simulink model "chap05"  (R2021a)
settings: Solver=FixedStepDiscrete  StartTime=0.0  StopTime=inf  FixedStep=0.001  RelTol=1e-3
undefined symbols (not defined in the file): DiscIntNeverNeededParam, Header, Pose, X, Y, Z
libraries: robotlib x31
(part 2 of 9)

== system chap05/Subsystem16/Subsystem1 ==
  In19 : Inport
  switch : Inport  Port=2
  Bus Creator : BusCreator  Inputs=3
  Bus Selector : BusSelector  OutputSignals=state(tk).node5.xx,state(tk).node5.xx0,state(tk).node3.xx,state(tk).node4.xx,state(tk).node5.vx,state(tk).node5.vx0,state(tk).node3.vx,state(tk).node4.vx
  Bus Selector1 : BusSelector  OutputSignals=state(tk).node5.xy,state(tk).node5.xy0,state(tk).node3.xy,state(tk).node4.xy,state(tk).node5.vy,state(tk).node5.vy0,state(tk).node3.vy,state(tk).node4.vy
  Bus Selector2 : BusSelector  OutputSignals=state(tk).node5.xz,state(tk).node5.xz0,state(tk).node3.xz,state(tk).node4.xz,state(tk).node5.vz,state(tk).node5.vz0,state(tk).node3.vz,state(tk).node4.vz
  Bus Selector3 : BusSelector  OutputSignals=state(t).node5.vx,state(t).node0.vx
  Bus Selector4 : BusSelector  OutputSignals=state(t).node5.vy,state(t).node0.vx
  Bus Selector5 : BusSelector  OutputSignals=state(t).node5.vz,state(t).node0.vz
  Bus Selector6 : BusSelector  OutputSignals=state(t).node5.vx,state(t).node5.vy,state(t).node5.vz
  Bus Selector7 : BusSelector  OutputSignals=state(t).node5.vx,state(t).node5.vy,state(t).node5.vz
  Bus Selector8 : BusSelector  OutputSignals=control.node5.ux,control.node5.uy,control.node5.uz
  Subsystem1 : Subsystem
  Subsystem10 : Subsystem
  Subsystem11 : Subsystem
      settings: PortSchema="{\"entries\":[{\"content\":{\"sides\":[{\"content\":{\"connectorIds\":[\"In1\",\"In2\",\"In3\",\"In4\"]},\"type\":\"ConnectorPlacement.EquallySpacedRectSide\",\"uuid\":\"3c32f130-2df4-4697-80e9-267a8217898e\"},{\"content\":{\"connectorIds\":[\"Out1\"],\"side\":\"RIGHT\"},\"type\":\"ConnectorPlacement.EquallySpacedRectSide\",\"uuid\":\"840675a7-4714-440f-a6ce-75eff1b2763f\"},{\"content\":{\"connectorIds\":[\"In5\"],\"side\":\"TOP\"},\"type\":\"ConnectorPlacement.EquallySpacedRectSide\",\"uuid\":\"5c23af56-4ec3-4a39-a531-12998a0be3c8\"},{\"content\":{\"connectorIds\":[\"Out2\"],\"side\":\"BOTTOM\"},\"type\":\"ConnectorPlacement.EquallySpacedRectSide\",\"uuid\":\"31d953fb-65a0-42e9-a844-060de010f298\"}]},\"type\":\"ConnectorPlacement.EquallySpacedConnector\",\"uuid\":\"61b27aa3-5880-401e-bae3-4611093a191a\"}],\"packageUris\":[\"http://schema.mathworks.com/mf0/Connector/R2020b\"],\"version\":\"1.0\"}"
  Subsystem2 : Subsystem
  Subsystem3 : Subsystem
      settings: PortSchema="{\"entries\":[{\"content\":{\"sides\":[{\"content\":{\"connectorIds\":[\"In1\",\"In2\",\"In3\",\"In4\",\"In5\",\"In6\",\"In7\",\"In8\",\"In9\"]},\"type\":\"ConnectorPlacement.EquallySpacedRectSide\",\"uuid\":\"e02b19dc-feca-4a5f-b0a9-7b682689d3dc\"},{\"content\":{\"connectorIds\":[\"Out1\",\"Out2\",\"Out3\"],\"side\":\"RIGHT\"},\"type\":\"ConnectorPlacement.EquallySpacedRectSide\",\"uuid\":\"6cba16a1-1866-4332-a766-c6ecae75c00a\"},{\"content\":{\"connectorIds\":[],\"side\":\"TOP\"},\"type\":\"ConnectorPlacement.EquallySpacedRectSide\",\"uuid\":\"834934d8-ba7c-4cfc-8528-dda956d123e9\"},{\"content\":{\"connectorIds\":[\"In10\"],\"side\":\"BOTTOM\"},\"type\":\"ConnectorPlacement.EquallySpacedRectSide\",\"uuid\":\"a447ec2e-850c-49d1-98c5-4201d925b22c\"}]},\"type\":\"ConnectorPlacement.EquallySpacedConnector\",\"uuid\":\"dde62e81-0b86-43c6-8cdc-67ebf109c079\"}],\"packageUris\":[\"http://schema.mathworks.com/mf0/Connector/R2020b\"],\"version\":\"1.0\"}"
  Subsystem5 : Subsystem
      settings: PortSchema="{\"entries\":[{\"content\":{\"sides\":[{\"content\":{\"connectorIds\":[\"In1\",\"In2\",\"In3\",\"In4\"]},\"type\":\"ConnectorPlacement.EquallySpacedRectSide\",\"uuid\":\"3c32f130-2df4-4697-80e9-267a8217898e\"},{\"content\":{\"connectorIds\":[\"Out1\"],\"side\":\"RIGHT\"},\"type\":\"ConnectorPlacement.EquallySpacedRectSide\",\"uuid\":\"840675a7-4714-440f-a6ce-75eff1b2763f\"},{\"content\":{\"connectorIds\":[\"In5\"],\"side\":\"TOP\"},\"type\":\"ConnectorPlacement.EquallySpacedRectSide\",\"uuid\":\"5c23af56-4ec3-4a39-a531-12998a0be3c8\"},{\"content\":{\"connectorIds\":[\"Out2\"],\"side\":\"BOTTOM\"},\"type\":\"ConnectorPlacement.EquallySpacedRectSide\",\"uuid\":\"31d953fb-65a0-42e9-a844-060de010f298\"}]},\"type\":\"ConnectorPlacement.EquallySpacedConnector\",\"uuid\":\"61b27aa3-5880-401e-bae3-4611093a191a\"}],\"packageUris\":[\"http://schema.mathworks.com/mf0/Connector/R2020b\"],\"version\":\"1.0\"}"
  Subsystem6 : Subsystem
  Subsystem8 : Subsystem
      settings: PortSchema="{\"entries\":[{\"content\":{\"sides\":[{\"content\":{\"connectorIds\":[\"In1\",\"In2\",\"In3\",\"In4\",\"In5\",\"In6\"]},\"type\":\"ConnectorPlacement.EquallySpacedRectSide\",\"uuid\":\"6e2ae49e-f829-4a88-ba6d-12a1c984ff97\"},{\"content\":{\"connectorIds\":[\"Out1\"],\"side\":\"RIGHT\"},\"type\":\"ConnectorPlacement.EquallySpacedRectSide\",\"uuid\":\"1d02df48-94d5-4b75-9fdc-37bb62799324\"},{\"content\":{\"connectorIds\":[],\"side\":\"TOP\"},\"type\":\"ConnectorPlacement.EquallySpacedRectSide\",\"uuid\":\"e0c2a01b-94eb-432a-818f-b3ac4af71c3e\"},{\"content\":{\"connectorIds\":[\"In7\"],\"side\":\"BOTTOM\"},\"type\":\"ConnectorPlacement.EquallySpacedRectSide\",\"uuid\":\"1c8c54e5-1608-4962-a210-31f0a1951aa9\"}]},\"type\":\"ConnectorPlacement.EquallySpacedConnector\",\"uuid\":\"4e183442-7783-4f10-aa1a-c21f2f9b268a\"}],\"packageUris\":[\"http://schema.mathworks.com/mf0/Connector/R2020b\"],\"version\":\"1.0\"}"
  Subsystem9 : Subsystem
      settings: PortSchema="{\"entries\":[{\"content\":{\"sides\":[{\"content\":{\"connectorIds\":[\"In1\",\"In2\",\"In3\",\"In4\"]},\"type\":\"ConnectorPlacement.EquallySpacedRectSide\",\"uuid\":\"3c32f130-2df4-4697-80e9-267a8217898e\"},{\"content\":{\"connectorIds\":[\"Out1\"],\"side\":\"RIGHT\"},\"type\":\"ConnectorPlacement.EquallySpacedRectSide\",\"uuid\":\"840675a7-4714-440f-a6ce-75eff1b2763f\"},{\"content\":{\"connectorIds\":[\"In5\"],\"side\":\"TOP\"},\"type\":\"ConnectorPlacement.EquallySpacedRectSide\",\"uuid\":\"5c23af56-4ec3-4a39-a531-12998a0be3c8\"},{\"content\":{\"connectorIds\":[\"Out2\"],\"side\":\"BOTTOM\"},\"type\":\"ConnectorPlacement.EquallySpacedRectSide\",\"uuid\":\"31d953fb-65a0-42e9-a844-060de010f298\"}]},\"type\":\"ConnectorPlacement.EquallySpacedConnector\",\"uuid\":\"61b27aa3-5880-401e-bae3-4611093a191a\"}],\"packageUris\":[\"http://schema.mathworks.com/mf0/Connector/R2020b\"],\"version\":\"1.0\"}"
  u5 : Outport
  wires:
  Bus Creator/1 -> u5/1  "node5"
  Bus Selector/5 -> Subsystem6/5(vx5)  "<vx>"
  Bus Selector/1 -> Subsystem6/1(xx5)  "<xx>"
  Bus Selector/3 -> Subsystem6/3(xx3)  "<xx>"
  Bus Selector/8 -> Subsystem6/8(vx4)  "<vx>"
  Bus Selector/7 -> Subsystem6/7(vx3)  "<vx>"
  Bus Selector/4 -> Subsystem6/4(xx4)  "<xx>"
  Bus Selector6/3 -> Subsystem8/6(vz)  "<vz>"
  Bus Selector6/1 -> Subsystem8/4(vx)  "<vx>"
  [Sx] -> Subsystem8/1(Sx)
  [Sz] -> Subsystem8/3(Sz)
  Subsystem8/1(" gain") -> [gain]  "p5"
  In19/1 -> [state], Bus Selector2/1, Bus Selector/1, Bus Selector1/1
  [state] -> Bus Selector6/1
  [Sy] -> Subsystem8/2(Sy)
  Bus Selector6/2 -> Subsystem8/5(vy)  "<vy>"
  Subsystem10/3(uz) -> Bus Creator/3  "uz"
  Subsystem10/2(uy) -> Bus Creator/2  "uy"
  Subsystem10/1(ux) -> Bus Creator/1  "ux"
  [state] -> Bus Selector7/1
  Bus Selector8/1 -> Subsystem3/6(ux)  "<ux>"
  Bus Selector7/2 -> Subsystem3/3(vy)  "<vy>"
  Bus Selector8/2 -> Subsystem3/7(uy)  "<uy>"
  [state] -> Bus Selector8/1
  Bus Selector7/1 -> Subsystem3/2(vx)  "<vx>"
  Bus Selector7/3 -> Subsystem3/4(vz)  "<vz>"
  Bus Selector8/3 -> Subsystem3/8(uz)  "<uz>"
  Subsystem3/1(udtx) -> Subsystem10/1(utx)
  Subsystem3/2(udty) -> Subsystem10/2(uty)
  Subsystem3/3(udtz) -> Subsystem10/3(utz)
  Bus Selector/2 -> Subsystem6/2(xx0)  "<xx0>"
  Bus Selector/6 -> Subsystem6/6(vx0)  "<vx0>"
  Bus Selector1/1 -> Subsystem1/1(xy5)  "<xy>"
  Bus Selector1/2 -> Subsystem1/2(xy0)  "<xy0>"
  Bus Selector1/3 -> Subsystem1/3(xy3)  "<xy>"
  Bus Selector1/4 -> Subsystem1/4(xy4)  "<xy>"
  Bus Selector1/5 -> Subsystem1/5(vy5)  "<vy>"
  Bus Selector1/6 -> Subsystem1/6(vy0)  "<vy0>"
  Bus Selector1/7 -> Subsystem1/7(vy3)  "<vy>"
  Bus Selector1/8 -> Subsystem1/8(vy4)  "<vy>"
  Bus Selector2/1 -> Subsystem2/1(xz5)  "<xz>"
  Bus Selector2/2 -> Subsystem2/2(xz0)  "<xz0>"
  Bus Selector2/3 -> Subsystem2/3(xz3)  "<xz>"
  Bus Selector2/4 -> Subsystem2/4(xz4)  "<xz>"
  Bus Selector2/5 -> Subsystem2/5(vz5)  "<vz>"
  Bus Selector2/6 -> Subsystem2/6(vz0)  "<vz0>"
  Bus Selector2/7 -> Subsystem2/7(vz3)  "<vz>"
  Bus Selector2/8 -> Subsystem2/8(vz4)  "<vz>"
  [gain] -> Subsystem11/4(gain)
  Subsystem9/1(uy) -> Subsystem3/5(uty)
  Subsystem2/1(utz) -> Subsystem11/3(utz)
  Subsystem1/1(uty) -> Subsystem9/3(uty)
  [state] -> Bus Selector3/1
  Subsystem5/1(ux) -> Subsystem3/1(utx)
  Bus Selector3/2 -> Subsystem5/2(vx0)  "<vx>"
  Bus Selector3/1 -> Subsystem5/1(vx5)  "<vx>"
  Subsystem11/1(uz) -> Subsystem3/9(utz)
  Bus Selector5/1 -> Subsystem11/1(vz5)  "<vz>"
  [state] -> Bus Selector4/1
  Subsystem6/1(utx) -> Subsystem5/3(utx)
  [state] -> Bus Selector5/1
  Bus Selector4/1 -> Subsystem9/1(vy5)  "<vy>"
  Bus Selector4/2 -> Subsystem9/2(vy0)  "<vx>"
  Bus Selector5/2 -> Subsystem11/2(vz0)  "<vz>"
  [gain] -> Subsystem5/4(gain)
  Subsystem5/2(Sx) -> [Sx]
  Subsystem9/2(Sz) -> [Sy]
  Subsystem11/2(Sz) -> [Sz]
  [gain] -> Subsystem9/4(gain)
  switch/1 -> [switch], Subsystem5/5(switch)
  [switch] -> Subsystem11/5(switch)
  [switch] -> Subsystem9/5(switch)
  [switch] -> Subsystem8/7(switch)
  [switch] -> Subsystem3/10(switch)

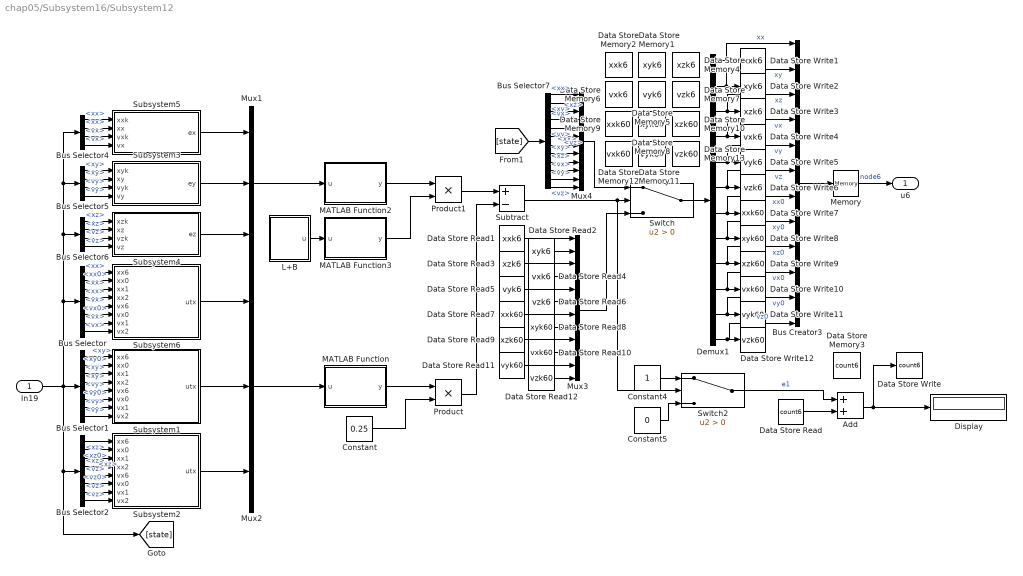
== system chap05/Subsystem16/Subsystem12 ==
  In19 : Inport
  Add : Sum
  Bus Creator3 : BusCreator  Inputs=12
  Bus Selector : BusSelector  OutputSignals=state(tk).node6.xx,state(tk).node6.xx0,state(tk).node1.xx,state(tk).node2.xx,state(tk).node6.vx,state(tk).node6.vx0,state(tk).node1.vx,state(tk).node2.vx
  Bus Selector1 : BusSelector  OutputSignals=state(tk).node6.xy,state(tk).node6.xy0,state(tk).node1.xy,state(tk).node2.xy,state(tk).node6.vy,state(tk).node6.vy0,state(tk).node1.vy,state(tk).node2.vy
  Bus Selector2 : BusSelector  OutputSignals=state(tk).node6.xz,state(tk).node6.xz0,state(tk).node1.xz,state(tk).node2.xz,state(tk).node6.vz,state(tk).node6.vz0,state(tk).node1.vz,state(tk).node2.vz
  Bus Selector4 : BusSelector  OutputSignals=state(tk).node6.xx,state(t).node6.xx,state(tk).node6.vx,state(t).node6.vx
  Bus Selector5 : BusSelector  OutputSignals=state(tk).node6.xy,state(t).node6.xy,state(tk).node6.vy,state(t).node6.vy
  Bus Selector6 : BusSelector  OutputSignals=state(tk).node6.xz,state(t).node6.xz,state(tk).node6.vz,state(t).node6.vz
  Bus Selector7 : BusSelector  OutputSignals=state(t).node6.xx,state(t).node6.xy,state(t).node6.xz,state(t).node6.vx,state(t).node6.vy,state(t).node6.vz,state(t).node0.xx,state(t).node0.xy,state(t).node0.xz,state(t).node0.vx,state(t).node0.vy,state(t).node0.vz
  Constant : Constant  Value=0.25
  Constant4 : Constant
  Constant5 : Constant  Value=0
  Data Store Memory1 : DataStoreMemory  DataStoreName=xyk6  ReadBeforeWriteMsg=warning  WriteAfterWriteMsg=warning  WriteAfterReadMsg=warning  ShowAdditionalParam=off
  Data Store Memory10 : DataStoreMemory  DataStoreName=xzk60  ReadBeforeWriteMsg=warning  WriteAfterWriteMsg=warning  WriteAfterReadMsg=warning  ShowAdditionalParam=off
  Data Store Memory11 : DataStoreMemory  DataStoreName=vyk60  ReadBeforeWriteMsg=warning  WriteAfterWriteMsg=warning  WriteAfterReadMsg=warning  ShowAdditionalParam=off
  Data Store Memory12 : DataStoreMemory  DataStoreName=vxk60  ReadBeforeWriteMsg=warning  WriteAfterWriteMsg=warning  WriteAfterReadMsg=warning  ShowAdditionalParam=off
  Data Store Memory13 : DataStoreMemory  DataStoreName=vzk60  ReadBeforeWriteMsg=warning  WriteAfterWriteMsg=warning  WriteAfterReadMsg=warning  ShowAdditionalParam=off
  Data Store Memory2 : DataStoreMemory  DataStoreName=xxk6  ReadBeforeWriteMsg=warning  WriteAfterWriteMsg=warning  WriteAfterReadMsg=warning  ShowAdditionalParam=off
  Data Store Memory3 : DataStoreMemory  DataStoreName=count6  ReadBeforeWriteMsg=warning  WriteAfterWriteMsg=warning  WriteAfterReadMsg=warning  ShowAdditionalParam=off
  Data Store Memory4 : DataStoreMemory  DataStoreName=xzk6  ReadBeforeWriteMsg=warning  WriteAfterWriteMsg=warning  WriteAfterReadMsg=warning  ShowAdditionalParam=off
  Data Store Memory5 : DataStoreMemory  DataStoreName=vyk6  ReadBeforeWriteMsg=warning  WriteAfterWriteMsg=warning  WriteAfterReadMsg=warning  ShowAdditionalParam=off
  Data Store Memory6 : DataStoreMemory  DataStoreName=vxk6  ReadBeforeWriteMsg=warning  WriteAfterWriteMsg=warning  WriteAfterReadMsg=warning  ShowAdditionalParam=off
  Data Store Memory7 : DataStoreMemory  DataStoreName=vzk6  ReadBeforeWriteMsg=warning  WriteAfterWriteMsg=warning  WriteAfterReadMsg=warning  ShowAdditionalParam=off
  Data Store Memory8 : DataStoreMemory  DataStoreName=xyk60  ReadBeforeWriteMsg=warning  WriteAfterWriteMsg=warning  WriteAfterReadMsg=warning  ShowAdditionalParam=off
  Data Store Memory9 : DataStoreMemory  DataStoreName=xxk60  ReadBeforeWriteMsg=warning  WriteAfterWriteMsg=warning  WriteAfterReadMsg=warning  ShowAdditionalParam=off
  Data Store Read : DataStoreRead  DataStoreName=count6  IndexOptions=Index vector (dialog)  Indices=1  OutputSizes=1
  Data Store Read1 : DataStoreRead  DataStoreName=xxk6  IndexOptions=Index vector (dialog)  Indices=1  OutputSizes=1
  Data Store Read10 : DataStoreRead  DataStoreName=vxk60  IndexOptions=Index vector (dialog)  Indices=1  OutputSizes=1
  Data Store Read11 : DataStoreRead  DataStoreName=vyk60  IndexOptions=Index vector (dialog)  Indices=1  OutputSizes=1
  Data Store Read12 : DataStoreRead  DataStoreName=vzk60  IndexOptions=Index vector (dialog)  Indices=1  OutputSizes=1
  Data Store Read2 : DataStoreRead  DataStoreName=xyk6  IndexOptions=Index vector (dialog)  Indices=1  OutputSizes=1
  Data Store Read3 : DataStoreRead  DataStoreName=xzk6  IndexOptions=Index vector (dialog)  Indices=1  OutputSizes=1
  Data Store Read4 : DataStoreRead  DataStoreName=vxk6  IndexOptions=Index vector (dialog)  Indices=1  OutputSizes=1
  Data Store Read5 : DataStoreRead  DataStoreName=vyk6  IndexOptions=Index vector (dialog)  Indices=1  OutputSizes=1
  Data Store Read6 : DataStoreRead  DataStoreName=vzk6  IndexOptions=Index vector (dialog)  Indices=1  OutputSizes=1
  Data Store Read7 : DataStoreRead  DataStoreName=xxk60  IndexOptions=Index vector (dialog)  Indices=1  OutputSizes=1
  Data Store Read8 : DataStoreRead  DataStoreName=xyk60  IndexOptions=Index vector (dialog)  Indices=1  OutputSizes=1
  Data Store Read9 : DataStoreRead  DataStoreName=xzk60  IndexOptions=Index vector (dialog)  Indices=1  OutputSizes=1
  Data Store Write : DataStoreWrite  DataStoreName=count6  IndexOptions=Index vector (dialog)  Indices=1  OutputSizes=1
  Data Store Write1 : DataStoreWrite  DataStoreName=xxk6  IndexOptions=Index vector (dialog)  Indices=1  OutputSizes=1
  Data Store Write10 : DataStoreWrite  DataStoreName=vxk60  IndexOptions=Index vector (dialog)  Indices=1  OutputSizes=1
  Data Store Write11 : DataStoreWrite  DataStoreName=vyk60  IndexOptions=Index vector (dialog)  Indices=1  OutputSizes=1
  Data Store Write12 : DataStoreWrite  DataStoreName=vzk60  IndexOptions=Index vector (dialog)  Indices=1  OutputSizes=1
  Data Store Write2 : DataStoreWrite  DataStoreName=xyk6  IndexOptions=Index vector (dialog)  Indices=1  OutputSizes=1
  Data Store Write3 : DataStoreWrite  DataStoreName=xzk6  IndexOptions=Index vector (dialog)  Indices=1  OutputSizes=1
  Data Store Write4 : DataStoreWrite  DataStoreName=vxk6  IndexOptions=Index vector (dialog)  Indices=1  OutputSizes=1
  Data Store Write5 : DataStoreWrite  DataStoreName=vyk6  IndexOptions=Index vector (dialog)  Indices=1  OutputSizes=1
  Data Store Write6 : DataStoreWrite  DataStoreName=vzk6  IndexOptions=Index vector (dialog)  Indices=1  OutputSizes=1
  Data Store Write7 : DataStoreWrite  DataStoreName=xxk60  IndexOptions=Index vector (dialog)  Indices=1  OutputSizes=1
  Data Store Write8 : DataStoreWrite  DataStoreName=xyk60  IndexOptions=Index vector (dialog)  Indices=1  OutputSizes=1
  Data Store Write9 : DataStoreWrite  DataStoreName=xzk60  IndexOptions=Index vector (dialog)  Indices=1  OutputSizes=1
  Demux1 : Demux  Outputs=12
  Display : Display
  L+B : Subsystem
  MATLAB Function : MATLAB Function  TreatAsAtomicUnit=on
  MATLAB Function2 : MATLAB Function  TreatAsAtomicUnit=on
  MATLAB Function3 : MATLAB Function  TreatAsAtomicUnit=on
  Memory : Memory
  Mux1 : Mux  Inputs=3
  Mux2 : Mux  Inputs=3
  Mux3 : Mux  Inputs=12
  Mux4 : Mux  Inputs=12
  Product : Product
  Product1 : Product
  Subsystem1 : Subsystem
  Subsystem2 : Subsystem
  Subsystem3 : Subsystem
  Subsystem4 : Subsystem
  Subsystem5 : Subsystem
  Subsystem6 : Subsystem
  Subtract : Sum  Inputs=+-
  Switch : Switch  Criteria=u2 > Threshold
  Switch2 : Switch  Criteria=u2 > Threshold
  u6 : Outport
  wires:
  Subsystem1/1(utx) -> Mux2/2
  Subsystem6/1(utx) -> Mux2/1
  Subsystem2/1(utx) -> Mux2/3
  Data Store Read/1 -> Add/2
  Subsystem3/1(ey) -> Mux1/2
  MATLAB Function/1(y) -> Product/1
  Mux2/1 -> MATLAB Function/1(u)
  Product1/1 -> Subtract/1
  Add/1 -> Data Store Write/1, Display/1
  Subsystem5/1(ex) -> Mux1/1
  Subsystem4/1(ez) -> Mux1/3
  Mux1/1 -> MATLAB Function2/1(u)
  L+B/1(u) -> MATLAB Function3/1(u)
  MATLAB Function2/1(y) -> Product1/1
  Constant4/1 -> Switch2/1
  Constant/1 -> Product/2
  Constant5/1 -> Switch2/3
  MATLAB Function3/1(y) -> Product1/2
  Switch2/1 -> Add/1  "e1"
  Product/1 -> Subtract/2
  Memory/1 -> u6/1  "node6"
  Bus Selector4/4 -> Subsystem5/4(vx)  "<vx>"
  Bus Selector5/3 -> Subsystem3/3(vyk)  "<vy>"
  Bus Selector5/2 -> Subsystem3/2(xy)  "<xy>"
  Bus Selector4/1 -> Subsystem5/1(xxk)  "<xx>"
  Bus Selector5/4 -> Subsystem3/4(vy)  "<vy>"
  Bus Selector5/1 -> Subsystem3/1(xyk)  "<xy>"
  In19/1 -> Bus Selector1/1, Bus Selector2/1, [state], Bus Selector/1, Bus Selector5/1, Bus Selector4/1, Bus Selector6/1
  Bus Selector4/3 -> Subsystem5/3(vxk)  "<vx>"
  Bus Selector6/2 -> Subsystem4/2(xz)  "<xz>"
  Bus Selector6/3 -> Subsystem4/3(vzk)  "<vz>"
  Bus Selector4/2 -> Subsystem5/2(xx)  "<xx>"
  Bus Selector6/4 -> Subsystem4/4(vz)  "<vz>"
  Bus Selector6/1 -> Subsystem4/1(xzk)  "<xz>"
  Subtract/1 -> Switch/2, Switch2/2
  Demux1/3 -> Data Store Write3/1, Bus Creator3/3  "xz"
  Demux1/12 -> Bus Creator3/12, Data Store Write12/1  "vz0"
  Demux1/9 -> Data Store Write9/1, Bus Creator3/9  "xz0"
  Data Store Read3/1 -> Mux3/3
  Bus Selector7/10 -> Mux4/10  "<vx>"
  Data Store Read2/1 -> Mux3/2
  Mux3/1 -> Switch/3
  Demux1/10 -> Data Store Write10/1, Bus Creator3/10  "vx0"
  Bus Selector7/5 -> Mux4/5  "<vy>"
  Data Store Read6/1 -> Mux3/6
  Data Store Read5/1 -> Mux3/5
  Demux1/5 -> Data Store Write5/1, Bus Creator3/5  "vy"
  Data Store Read1/1 -> Mux3/1
  Demux1/11 -> Data Store Write11/1, Bus Creator3/11  "vy0"
  Demux1/1 -> Data Store Write1/1, Bus Creator3/1  "xx"
  Data Store Read4/1 -> Mux3/4
  [state] -> Bus Selector7/1
  Data Store Read11/1 -> Mux3/11
  Demux1/6 -> Data Store Write6/1, Bus Creator3/6  "vz"
  Bus Selector7/2 -> Mux4/2  "<xy>"
  Bus Selector7/1 -> Mux4/1  "<xx>"
  Bus Selector7/8 -> Mux4/8  "<xy>"
  Data Store Read10/1 -> Mux3/10
  Bus Selector7/4 -> Mux4/4  "<vx>"
  Mux4/1 -> Switch/1
  Data Store Read12/1 -> Mux3/12
  Bus Creator3/1 -> Memory/1
  Bus Selector7/7 -> Mux4/7  "<xx>"
  Bus Selector7/6 -> Mux4/6  "<vz>"
  Demux1/2 -> Data Store Write2/1, Bus Creator3/2  "xy"
  Demux1/4 -> Data Store Write4/1, Bus Creator3/4  "vx"
  Data Store Read9/1 -> Mux3/9
  Bus Selector7/11 -> Mux4/11  "<vy>"
  Bus Selector7/9 -> Mux4/9  "<xz>"
  Demux1/8 -> Data Store Write8/1, Bus Creator3/8  "xy0"
  Demux1/7 -> Data Store Write7/1, Bus Creator3/7  "xx0"
  Bus Selector7/3 -> Mux4/3  "<xz>"
  Data Store Read7/1 -> Mux3/7
  Data Store Read8/1 -> Mux3/8
  Switch/1 -> Demux1/1
  Bus Selector7/12 -> Mux4/12  "<vz>"
  Bus Selector/2 -> Subsystem6/2(xx0)  "<xx0>"
  Bus Selector1/4 -> Subsystem1/4(xx2)  "<xy>"
  Bus Selector/8 -> Subsystem6/8(vx2)  "<vx>"
  Bus Selector1/5 -> Subsystem1/5(vx6)  "<vy>"
  Bus Selector/6 -> Subsystem6/6(vx0)  "<vx0>"
  Bus Selector1/7 -> Subsystem1/7(vx1)  "<vy>"
  Bus Selector1/2 -> Subsystem1/2(xx0)  "<xy0>"
  Bus Selector1/1 -> Subsystem1/1(xx6)  "<xy>"
  Bus Selector2/1 -> Subsystem2/1(xx6)  "<xz>"
  Bus Selector2/6 -> Subsystem2/6(vx0)  "<vz0>"
  Bus Selector2/5 -> Subsystem2/5(vx6)  "<vz>"
  Bus Selector/5 -> Subsystem6/5(vx6)  "<vx>"
  Bus Selector/7 -> Subsystem6/7(vx1)  "<vx>"
  Bus Selector1/8 -> Subsystem1/8(vx2)  "<vy>"
  Bus Selector2/2 -> Subsystem2/2(xx0)  "<xz0>"
  Bus Selector2/4 -> Subsystem2/4(xx2)  "<xz>"
  Bus Selector/4 -> Subsystem6/4(xx2)  "<xx>"
  Bus Selector/1 -> Subsystem6/1(xx6)  "<xx>"
  Bus Selector1/6 -> Subsystem1/6(vx0)  "<vy0>"
  Bus Selector1/3 -> Subsystem1/3(xx1)  "<xy>"
  Bus Selector/3 -> Subsystem6/3(xx1)  "<xx>"
  Bus Selector2/3 -> Subsystem2/3(xx1)  "<xz>"
  Bus Selector2/7 -> Subsystem2/7(vx1)  "<vz>"
  Bus Selector2/8 -> Subsystem2/8(vx2)  "<vz>"

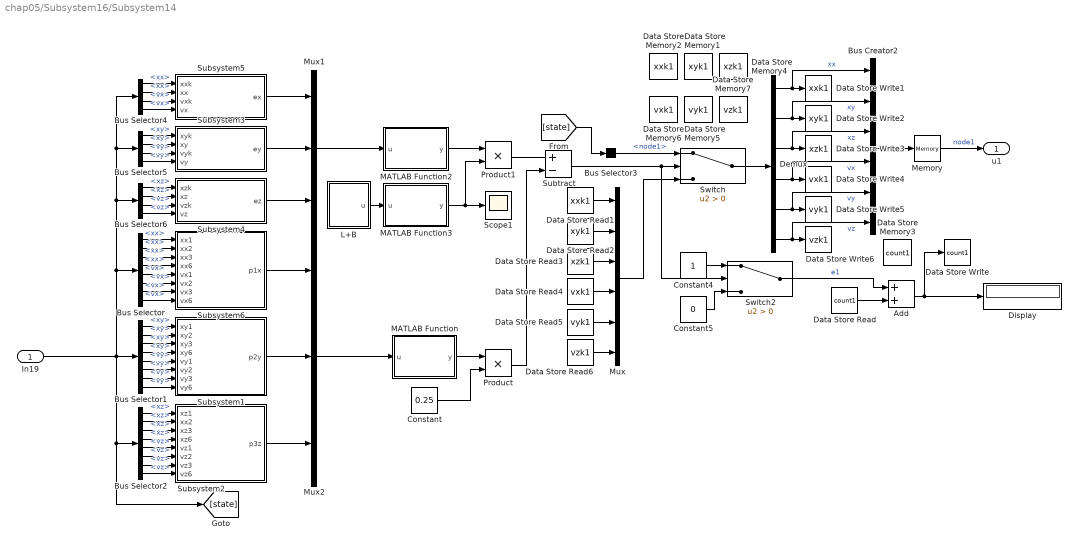
== system chap05/Subsystem16/Subsystem14 ==
  In19 : Inport
  Add : Sum
  Bus Creator2 : BusCreator  Inputs=6
  Bus Selector : BusSelector  OutputSignals=state(tk).node1.xx,state(tk).node2.xx,state(tk).node3.xx,state(tk).node6.xx,state(tk).node1.vx,state(tk).node2.vx,state(tk).node3.vx,state(tk).node6.vx
  Bus Selector1 : BusSelector  OutputSignals=state(tk).node1.xy,state(tk).node2.xy,state(tk).node3.xy,state(tk).node6.xy,state(tk).node1.vy,state(tk).node2.vy,state(tk).node3.vy,state(tk).node6.vy
  Bus Selector2 : BusSelector  OutputSignals=state(tk).node1.xz,state(tk).node2.xz,state(tk).node3.xz,state(tk).node6.xz,state(tk).node1.vz,state(tk).node2.vz,state(tk).node3.vz,state(tk).node6.vz
  Bus Selector3 : BusSelector  OutputSignals=state(t).node1
  Bus Selector4 : BusSelector  OutputSignals=state(tk).node1.xx,state(t).node1.xx,state(tk).node1.vx,state(t).node1.vx
  Bus Selector5 : BusSelector  OutputSignals=state(tk).node1.xy,state(t).node1.xy,state(tk).node1.vy,state(t).node1.vy
  Bus Selector6 : BusSelector  OutputSignals=state(tk).node1.xz,state(t).node1.xz,state(tk).node1.vz,state(t).node1.vz
  Constant : Constant  Value=0.25
  Constant4 : Constant
  Constant5 : Constant  Value=0
  Data Store Memory1 : DataStoreMemory  DataStoreName=xyk1  ReadBeforeWriteMsg=warning  WriteAfterWriteMsg=warning  WriteAfterReadMsg=warning  ShowAdditionalParam=off
  Data Store Memory2 : DataStoreMemory  DataStoreName=xxk1  ReadBeforeWriteMsg=warning  WriteAfterWriteMsg=warning  WriteAfterReadMsg=warning  ShowAdditionalParam=off
  Data Store Memory3 : DataStoreMemory  DataStoreName=count1  ReadBeforeWriteMsg=warning  WriteAfterWriteMsg=warning  WriteAfterReadMsg=warning  ShowAdditionalParam=off
  Data Store Memory4 : DataStoreMemory  DataStoreName=xzk1  ReadBeforeWriteMsg=warning  WriteAfterWriteMsg=warning  WriteAfterReadMsg=warning  ShowAdditionalParam=off
  Data Store Memory5 : DataStoreMemory  DataStoreName=vyk1  ReadBeforeWriteMsg=warning  WriteAfterWriteMsg=warning  WriteAfterReadMsg=warning  ShowAdditionalParam=off
  Data Store Memory6 : DataStoreMemory  DataStoreName=vxk1  ReadBeforeWriteMsg=warning  WriteAfterWriteMsg=warning  WriteAfterReadMsg=warning  ShowAdditionalParam=off
  Data Store Memory7 : DataStoreMemory  DataStoreName=vzk1  ReadBeforeWriteMsg=warning  WriteAfterWriteMsg=warning  WriteAfterReadMsg=warning  ShowAdditionalParam=off
  Data Store Read : DataStoreRead  DataStoreName=count1  IndexOptions=Index vector (dialog)  Indices=1  OutputSizes=1
  Data Store Read1 : DataStoreRead  DataStoreName=xxk1  IndexOptions=Index vector (dialog)  Indices=1  OutputSizes=1
  Data Store Read2 : DataStoreRead  DataStoreName=xyk1  IndexOptions=Index vector (dialog)  Indices=1  OutputSizes=1
  Data Store Read3 : DataStoreRead  DataStoreName=xzk1  IndexOptions=Index vector (dialog)  Indices=1  OutputSizes=1
  Data Store Read4 : DataStoreRead  DataStoreName=vxk1  IndexOptions=Index vector (dialog)  Indices=1  OutputSizes=1
  Data Store Read5 : DataStoreRead  DataStoreName=vyk1  IndexOptions=Index vector (dialog)  Indices=1  OutputSizes=1
  Data Store Read6 : DataStoreRead  DataStoreName=vzk1  IndexOptions=Index vector (dialog)  Indices=1  OutputSizes=1
  Data Store Write : DataStoreWrite  DataStoreName=count1  IndexOptions=Index vector (dialog)  Indices=1  OutputSizes=1
  Data Store Write1 : DataStoreWrite  DataStoreName=xxk1  IndexOptions=Index vector (dialog)  Indices=1  OutputSizes=1
  Data Store Write2 : DataStoreWrite  DataStoreName=xyk1  IndexOptions=Index vector (dialog)  Indices=1  OutputSizes=1
  Data Store Write3 : DataStoreWrite  DataStoreName=xzk1  IndexOptions=Index vector (dialog)  Indices=1  OutputSizes=1
  Data Store Write4 : DataStoreWrite  DataStoreName=vxk1  IndexOptions=Index vector (dialog)  Indices=1  OutputSizes=1
  Data Store Write5 : DataStoreWrite  DataStoreName=vyk1  IndexOptions=Index vector (dialog)  Indices=1  OutputSizes=1
  Data Store Write6 : DataStoreWrite  DataStoreName=vzk1  IndexOptions=Index vector (dialog)  Indices=1  OutputSizes=1
  Demux : Demux  Outputs=6
  Display : Display
  L+B : Subsystem
  MATLAB Function : MATLAB Function  TreatAsAtomicUnit=on
  MATLAB Function2 : MATLAB Function  TreatAsAtomicUnit=on
  MATLAB Function3 : MATLAB Function  TreatAsAtomicUnit=on
  Memory : Memory
  Mux : Mux  Inputs=6
  Mux1 : Mux  Inputs=3
  Mux2 : Mux  Inputs=3
  Product : Product
  Product1 : Product
  Scope1 : Scope
  Subsystem1 : Subsystem
  Subsystem2 : Subsystem
  Subsystem3 : Subsystem
  Subsystem4 : Subsystem
  Subsystem5 : Subsystem
  Subsystem6 : Subsystem
  Subtract : Sum  Inputs=+-
  Switch : Switch  Criteria=u2 > Threshold
  Switch2 : Switch  Criteria=u2 > Threshold
  u1 : Outport
  wires:
  Bus Selector2/8 -> Subsystem2/8(vz6)  "<vz>"
  Bus Selector2/7 -> Subsystem2/7(vz3)  "<vz>"
  Bus Selector2/6 -> Subsystem2/6(vz2)  "<vz>"
  Bus Selector2/5 -> Subsystem2/5(vz1)  "<vz>"
  Bus Selector2/4 -> Subsystem2/4(xz6)  "<xz>"
  Bus Selector2/3 -> Subsystem2/3(xz3)  "<xz>"
  Bus Selector2/2 -> Subsystem2/2(xx2)  "<xz>"
  Bus Selector2/1 -> Subsystem2/1(xz1)  "<xz>"
  Bus Selector1/8 -> Subsystem1/8(vy6)  "<vy>"
  Bus Selector1/7 -> Subsystem1/7(vy3)  "<vy>"
  Bus Selector1/6 -> Subsystem1/6(vy2)  "<vy>"
  Bus Selector1/5 -> Subsystem1/5(vy1)  "<vy>"
  Bus Selector1/4 -> Subsystem1/4(xy6)  "<xy>"
  Bus Selector1/3 -> Subsystem1/3(xy3)  "<xy>"
  Bus Selector1/2 -> Subsystem1/2(xy2)  "<xy>"
  Bus Selector1/1 -> Subsystem1/1(xy1)  "<xy>"
  Bus Selector/8 -> Subsystem6/8(vx6)  "<vx>"
  Bus Selector/7 -> Subsystem6/7(vx3)  "<vx>"
  Bus Selector/6 -> Subsystem6/6(vx2)  "<vx>"
  Bus Selector/5 -> Subsystem6/5(vx1)  "<vx>"
  Bus Selector/4 -> Subsystem6/4(xx6)  "<xx>"
  Bus Selector/3 -> Subsystem6/3(xx3)  "<xx>"
  Bus Selector/2 -> Subsystem6/2(xx2)  "<xx>"
  Bus Selector/1 -> Subsystem6/1(xx1)  "<xx>"
  Mux2/1 -> MATLAB Function/1(u)
  Subsystem1/1(p2y) -> Mux2/2
  Subsystem6/1(p1x) -> Mux2/1
  Subsystem2/1(p3z) -> Mux2/3
  MATLAB Function/1(y) -> Product/1
  Constant/1 -> Product/2
  Subsystem4/1(ez) -> Mux1/3
  Subsystem5/1(ex) -> Mux1/1
  Subsystem3/1(ey) -> Mux1/2
  Mux1/1 -> MATLAB Function2/1(u)
  MATLAB Function2/1(y) -> Product1/1
  L+B/1(u) -> MATLAB Function3/1(u)
  MATLAB Function3/1(y) -> Product1/2, Scope1/1
  Memory/1 -> u1/1  "node1"
  Data Store Read5/1 -> Mux/5
  Data Store Read/1 -> Add/2
  Product1/1 -> Subtract/1
  Add/1 -> Display/1, Data Store Write/1
  Mux/1 -> Switch/3
  Constant4/1 -> Switch2/1
  Data Store Read3/1 -> Mux/3
  Data Store Read1/1 -> Mux/1
  Bus Selector3/1 -> Switch/1  "<node1>"
  Constant5/1 -> Switch2/3
  Switch2/1 -> Add/1  "e1"
  Data Store Read6/1 -> Mux/6
  Switch/1 -> Demux/1
  Data Store Read2/1 -> Mux/2
  Data Store Read4/1 -> Mux/4
  Product/1 -> Subtract/2
  [state] -> Bus Selector3/1
  Demux/1 -> Bus Creator2/1, Data Store Write1/1  "xx"
  Demux/2 -> Bus Creator2/2, Data Store Write2/1  "xy"
  Demux/3 -> Bus Creator2/3, Data Store Write3/1  "xz"
  Demux/4 -> Bus Creator2/4, Data Store Write4/1  "vx"
  Demux/5 -> Bus Creator2/5, Data Store Write5/1  "vy"
  Demux/6 -> Bus Creator2/6, Data Store Write6/1  "vz"
  In19/1 -> [state], Bus Selector2/1, Bus Selector/1, Bus Selector6/1, Bus Selector5/1, Bus Selector4/1, Bus Selector1/1
  Bus Selector6/1 -> Subsystem4/1(xzk)  "<xz>"
  Bus Selector6/2 -> Subsystem4/2(xz)  "<xz>"
  Bus Selector6/3 -> Subsystem4/3(vzk)  "<vz>"
  Bus Selector6/4 -> Subsystem4/4(vz)  "<vz>"
  Bus Selector4/3 -> Subsystem5/3(vxk)  "<vx>"
  Bus Selector4/2 -> Subsystem5/2(xx)  "<xx>"
  Bus Selector4/1 -> Subsystem5/1(xxk)  "<xx>"
  Bus Selector4/4 -> Subsystem5/4(vx)  "<vx>"
  Bus Selector5/1 -> Subsystem3/1(xyk)  "<xy>"
  Bus Selector5/2 -> Subsystem3/2(xy)  "<xy>"
  Bus Selector5/3 -> Subsystem3/3(vyk)  "<vy>"
  Bus Selector5/4 -> Subsystem3/4(vy)  "<vy>"
  Bus Creator2/1 -> Memory/1
  Subtract/1 -> Switch/2, Switch2/2

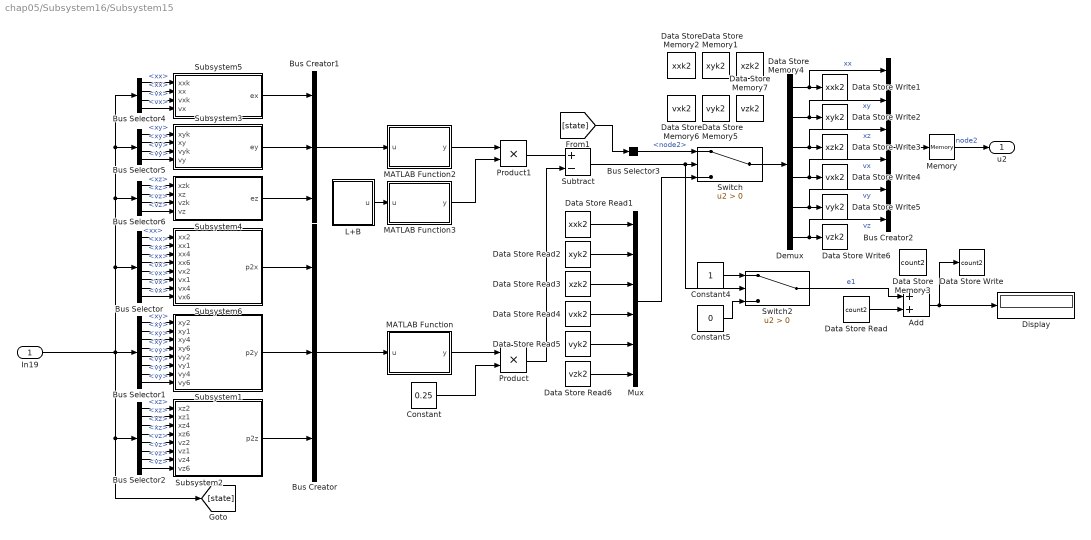
== system chap05/Subsystem16/Subsystem15 ==
  In19 : Inport
  Add : Sum
  Bus Creator : BusCreator  Inputs=3
  Bus Creator1 : BusCreator  Inputs=3
  Bus Creator2 : BusCreator  Inputs=6
  Bus Selector : BusSelector  OutputSignals=state(tk).node2.xx,state(tk).node1.xx,state(tk).node4.xx,state(tk).node6.xx,state(tk).node2.vx,state(tk).node1.vx,state(tk).node4.vx,state(tk).node6.vx
  Bus Selector1 : BusSelector  OutputSignals=state(tk).node2.xy,state(tk).node1.xy,state(tk).node4.xy,state(tk).node6.xy,state(tk).node2.vy,state(tk).node1.vy,state(tk).node4.vy,state(tk).node6.vy
  Bus Selector2 : BusSelector  OutputSignals=state(tk).node2.xz,state(tk).node1.xz,state(tk).node4.xz,state(tk).node6.xz,state(tk).node2.vz,state(tk).node1.vz,state(tk).node4.vz,state(tk).node6.vz
  Bus Selector3 : BusSelector  OutputSignals=state(t).node2
  Bus Selector4 : BusSelector  OutputSignals=state(tk).node2.xx,state(t).node2.xx,state(tk).node2.vx,state(t).node2.vx
  Bus Selector5 : BusSelector  OutputSignals=state(tk).node2.xy,state(t).node2.xy,state(tk).node2.vy,state(t).node2.vy
  Bus Selector6 : BusSelector  OutputSignals=state(tk).node2.xz,state(t).node2.xz,state(tk).node2.vz,state(t).node2.vz
  Constant : Constant  Value=0.25
  Constant4 : Constant
  Constant5 : Constant  Value=0
  Data Store Memory1 : DataStoreMemory  DataStoreName=xyk2  ReadBeforeWriteMsg=warning  WriteAfterWriteMsg=warning  WriteAfterReadMsg=warning  ShowAdditionalParam=off
  Data Store Memory2 : DataStoreMemory  DataStoreName=xxk2  ReadBeforeWriteMsg=warning  WriteAfterWriteMsg=warning  WriteAfterReadMsg=warning  ShowAdditionalParam=off
  Data Store Memory3 : DataStoreMemory  DataStoreName=count2  ReadBeforeWriteMsg=warning  WriteAfterWriteMsg=warning  WriteAfterReadMsg=warning  ShowAdditionalParam=off
  Data Store Memory4 : DataStoreMemory  DataStoreName=xzk2  ReadBeforeWriteMsg=warning  WriteAfterWriteMsg=warning  WriteAfterReadMsg=warning  ShowAdditionalParam=off
  Data Store Memory5 : DataStoreMemory  DataStoreName=vyk2  ReadBeforeWriteMsg=warning  WriteAfterWriteMsg=warning  WriteAfterReadMsg=warning  ShowAdditionalParam=off
  Data Store Memory6 : DataStoreMemory  DataStoreName=vxk2  ReadBeforeWriteMsg=warning  WriteAfterWriteMsg=warning  WriteAfterReadMsg=warning  ShowAdditionalParam=off
  Data Store Memory7 : DataStoreMemory  DataStoreName=vzk2  ReadBeforeWriteMsg=warning  WriteAfterWriteMsg=warning  WriteAfterReadMsg=warning  ShowAdditionalParam=off
  Data Store Read : DataStoreRead  DataStoreName=count2  IndexOptions=Index vector (dialog)  Indices=1  OutputSizes=1
  Data Store Read1 : DataStoreRead  DataStoreName=xxk2  IndexOptions=Index vector (dialog)  Indices=1  OutputSizes=1
  Data Store Read2 : DataStoreRead  DataStoreName=xyk2  IndexOptions=Index vector (dialog)  Indices=1  OutputSizes=1
  Data Store Read3 : DataStoreRead  DataStoreName=xzk2  IndexOptions=Index vector (dialog)  Indices=1  OutputSizes=1
  Data Store Read4 : DataStoreRead  DataStoreName=vxk2  IndexOptions=Index vector (dialog)  Indices=1  OutputSizes=1
  Data Store Read5 : DataStoreRead  DataStoreName=vyk2  IndexOptions=Index vector (dialog)  Indices=1  OutputSizes=1
  Data Store Read6 : DataStoreRead  DataStoreName=vzk2  IndexOptions=Index vector (dialog)  Indices=1  OutputSizes=1
  Data Store Write : DataStoreWrite  DataStoreName=count2  IndexOptions=Index vector (dialog)  Indices=1  OutputSizes=1
  Data Store Write1 : DataStoreWrite  DataStoreName=xxk2  IndexOptions=Index vector (dialog)  Indices=1  OutputSizes=1
  Data Store Write2 : DataStoreWrite  DataStoreName=xyk2  IndexOptions=Index vector (dialog)  Indices=1  OutputSizes=1
  Data Store Write3 : DataStoreWrite  DataStoreName=xzk2  IndexOptions=Index vector (dialog)  Indices=1  OutputSizes=1
  Data Store Write4 : DataStoreWrite  DataStoreName=vxk2  IndexOptions=Index vector (dialog)  Indices=1  OutputSizes=1
  Data Store Write5 : DataStoreWrite  DataStoreName=vyk2  IndexOptions=Index vector (dialog)  Indices=1  OutputSizes=1
  Data Store Write6 : DataStoreWrite  DataStoreName=vzk2  IndexOptions=Index vector (dialog)  Indices=1  OutputSizes=1
  Demux : Demux  Outputs=6
  Display : Display
  L+B : Subsystem
  MATLAB Function : MATLAB Function  TreatAsAtomicUnit=on
  MATLAB Function2 : MATLAB Function  TreatAsAtomicUnit=on
  MATLAB Function3 : MATLAB Function  TreatAsAtomicUnit=on
  Memory : Memory
  Mux : Mux  Inputs=6
  Product : Product
  Product1 : Product
  Subsystem1 : Subsystem
  Subsystem2 : Subsystem
  Subsystem3 : Subsystem
  Subsystem4 : Subsystem
  Subsystem5 : Subsystem
  Subsystem6 : Subsystem
  Subtract : Sum  Inputs=+-
  Switch : Switch  Criteria=u2 > Threshold
  Switch2 : Switch  Criteria=u2 > Threshold
  u2 : Outport
  wires:
  Bus Selector2/8 -> Subsystem2/8(vz6)  "<vz>"
  Bus Selector2/7 -> Subsystem2/7(vz4)  "<vz>"
  Bus Selector2/6 -> Subsystem2/6(vz1)  "<vz>"
  Bus Selector2/5 -> Subsystem2/5(vz2)  "<vz>"
  Bus Selector2/4 -> Subsystem2/4(xz6)  "<xz>"
  Bus Selector2/3 -> Subsystem2/3(xz4)  "<xz>"
  Bus Selector2/2 -> Subsystem2/2(xz1)  "<xz>"
  Bus Selector2/1 -> Subsystem2/1(xz2)  "<xz>"
  Bus Selector1/8 -> Subsystem1/8(vy6)  "<vy>"
  Bus Selector1/7 -> Subsystem1/7(vy4)  "<vy>"
  Bus Selector1/6 -> Subsystem1/6(vy1)  "<vy>"
  Bus Selector1/5 -> Subsystem1/5(vy2)  "<vy>"
  Bus Selector1/4 -> Subsystem1/4(xy6)  "<xy>"
  Bus Selector1/3 -> Subsystem1/3(xy4)  "<xy>"
  Bus Selector1/2 -> Subsystem1/2(xy1)  "<xy>"
  Bus Selector1/1 -> Subsystem1/1(xy2)  "<xy>"
  Bus Selector/8 -> Subsystem6/8(vx6)  "<vx>"
  Bus Selector/7 -> Subsystem6/7(vx4)  "<vx>"
  Bus Selector/6 -> Subsystem6/6(vx1)  "<vx>"
  Bus Selector/5 -> Subsystem6/5(vx2)  "<vx>"
  Bus Selector/4 -> Subsystem6/4(xx6)  "<xx>"
  Bus Selector/3 -> Subsystem6/3(xx4)  "<xx>"
  Bus Selector/2 -> Subsystem6/2(xx1)  "<xx>"
  Bus Selector/1 -> Subsystem6/1(xx2)  "<xx>"
  Subsystem2/1(p2z) -> Bus Creator/3
  Subsystem6/1(p2x) -> Bus Creator/1
  Subsystem1/1(p2y) -> Bus Creator/2
  Subsystem3/1(ey) -> Bus Creator1/2
  Subsystem4/1(ez) -> Bus Creator1/3
  MATLAB Function3/1(y) -> Product1/2
  Constant/1 -> Product/2
  MATLAB Function2/1(y) -> Product1/1
  MATLAB Function/1(y) -> Product/1
  Subsystem5/1(ex) -> Bus Creator1/1
  Bus Creator1/1 -> MATLAB Function2/1(u)
  Bus Creator/1 -> MATLAB Function/1(u)
  Data Store Read5/1 -> Mux/5
  Data Store Read/1 -> Add/2
  Product1/1 -> Subtract/1
  Add/1 -> Data Store Write/1, Display/1
  Mux/1 -> Switch/3
  Constant4/1 -> Switch2/1
  Data Store Read3/1 -> Mux/3
  Data Store Read1/1 -> Mux/1
  Bus Selector3/1 -> Switch/1  "<node2>"
  Constant5/1 -> Switch2/3
  Switch2/1 -> Add/1  "e1"
  Data Store Read6/1 -> Mux/6
  Switch/1 -> Demux/1
  Data Store Read2/1 -> Mux/2
  Data Store Read4/1 -> Mux/4
  Product/1 -> Subtract/2
  [state] -> Bus Selector3/1
  Demux/2 -> Bus Creator2/2, Data Store Write2/1  "xy"
  Demux/1 -> Bus Creator2/1, Data Store Write1/1  "xx"
  Demux/5 -> Bus Creator2/5, Data Store Write5/1  "vy"
  Demux/6 -> Bus Creator2/6, Data Store Write6/1  "vz"
  Demux/3 -> Bus Creator2/3, Data Store Write3/1  "xz"
  Memory/1 -> u2/1  "node2"
  Demux/4 -> Bus Creator2/4, Data Store Write4/1  "vx"
  In19/1 -> [state], Bus Selector2/1, Bus Selector6/1, Bus Selector5/1, Bus Selector4/1, Bus Selector/1, Bus Selector1/1
  Bus Selector4/1 -> Subsystem5/1(xxk)  "<xx>"
  Bus Selector4/2 -> Subsystem5/2(xx)  "<xx>"
  Bus Selector4/3 -> Subsystem5/3(vxk)  "<vx>"
  Bus Selector4/4 -> Subsystem5/4(vx)  "<vx>"
  Bus Selector5/1 -> Subsystem3/1(xyk)  "<xy>"
  Bus Selector5/2 -> Subsystem3/2(xy)  "<xy>"
  Bus Selector5/3 -> Subsystem3/3(vyk)  "<vy>"
  Bus Selector5/4 -> Subsystem3/4(vy)  "<vy>"
  Bus Selector6/1 -> Subsystem4/1(xzk)  "<xz>"
  Bus Selector6/2 -> Subsystem4/2(xz)  "<xz>"
  Bus Selector6/3 -> Subsystem4/3(vzk)  "<vz>"
  Bus Selector6/4 -> Subsystem4/4(vz)  "<vz>"
  Bus Creator2/1 -> Memory/1
  Subtract/1 -> Switch/2, Switch2/2
  L+B/1(u) -> MATLAB Function3/1(u)

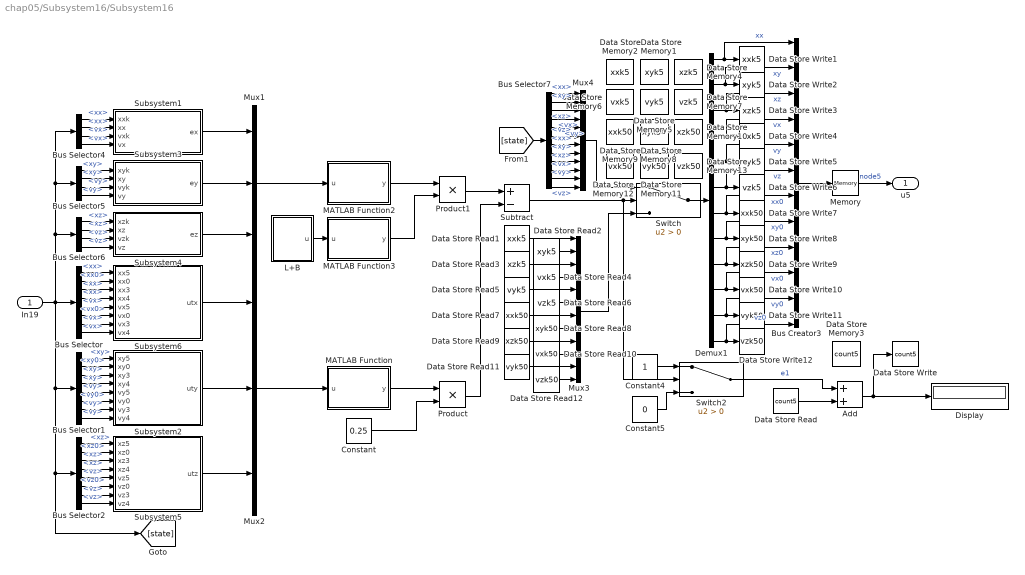
== system chap05/Subsystem16/Subsystem16 ==
  In19 : Inport
  Add : Sum
  Bus Creator3 : BusCreator  Inputs=12
  Bus Selector : BusSelector  OutputSignals=state(tk).node5.xx,state(tk).node5.xx0,state(tk).node3.xx,state(tk).node4.xx,state(tk).node5.vx,state(tk).node5.vx0,state(tk).node3.vx,state(tk).node4.vx
  Bus Selector1 : BusSelector  OutputSignals=state(tk).node5.xy,state(tk).node5.xy0,state(tk).node3.xy,state(tk).node4.xy,state(tk).node5.vy,state(tk).node5.vy0,state(tk).node3.vy,state(tk).node4.vy
  Bus Selector2 : BusSelector  OutputSignals=state(tk).node5.xz,state(tk).node5.xz0,state(tk).node3.xz,state(tk).node4.xz,state(tk).node5.vz,state(tk).node5.vz0,state(tk).node3.vz,state(tk).node4.vz
  Bus Selector4 : BusSelector  OutputSignals=state(tk).node5.xx,state(t).node5.xx,state(tk).node5.vx,state(t).node5.vx
  Bus Selector5 : BusSelector  OutputSignals=state(tk).node5.xy,state(t).node5.xy,state(tk).node5.vy,state(t).node5.vy
  Bus Selector6 : BusSelector  OutputSignals=state(tk).node5.xz,state(t).node5.xz,state(tk).node5.vz,state(t).node5.vz
  Bus Selector7 : BusSelector  OutputSignals=state(t).node5.xx,state(t).node5.xy,state(t).node5.xz,state(t).node5.vx,state(t).node5.vy,state(t).node5.vz,state(t).node0.xx,state(t).node0.xy,state(t).node0.xz,state(t).node0.vx,state(t).node0.vy,state(t).node0.vz
  Constant : Constant  Value=0.25
  Constant4 : Constant
  Constant5 : Constant  Value=0
  Data Store Memory1 : DataStoreMemory  DataStoreName=xyk5  ReadBeforeWriteMsg=warning  WriteAfterWriteMsg=warning  WriteAfterReadMsg=warning  ShowAdditionalParam=off
  Data Store Memory10 : DataStoreMemory  DataStoreName=xzk50  ReadBeforeWriteMsg=warning  WriteAfterWriteMsg=warning  WriteAfterReadMsg=warning  ShowAdditionalParam=off
  Data Store Memory11 : DataStoreMemory  DataStoreName=vyk50  ReadBeforeWriteMsg=warning  WriteAfterWriteMsg=warning  WriteAfterReadMsg=warning  ShowAdditionalParam=off
  Data Store Memory12 : DataStoreMemory  DataStoreName=vxk50  ReadBeforeWriteMsg=warning  WriteAfterWriteMsg=warning  WriteAfterReadMsg=warning  ShowAdditionalParam=off
  Data Store Memory13 : DataStoreMemory  DataStoreName=vzk50  ReadBeforeWriteMsg=warning  WriteAfterWriteMsg=warning  WriteAfterReadMsg=warning  ShowAdditionalParam=off
  Data Store Memory2 : DataStoreMemory  DataStoreName=xxk5  ReadBeforeWriteMsg=warning  WriteAfterWriteMsg=warning  WriteAfterReadMsg=warning  ShowAdditionalParam=off
  Data Store Memory3 : DataStoreMemory  DataStoreName=count5  ReadBeforeWriteMsg=warning  WriteAfterWriteMsg=warning  WriteAfterReadMsg=warning  ShowAdditionalParam=off
  Data Store Memory4 : DataStoreMemory  DataStoreName=xzk5  ReadBeforeWriteMsg=warning  WriteAfterWriteMsg=warning  WriteAfterReadMsg=warning  ShowAdditionalParam=off
  Data Store Memory5 : DataStoreMemory  DataStoreName=vyk5  ReadBeforeWriteMsg=warning  WriteAfterWriteMsg=warning  WriteAfterReadMsg=warning  ShowAdditionalParam=off
  Data Store Memory6 : DataStoreMemory  DataStoreName=vxk5  ReadBeforeWriteMsg=warning  WriteAfterWriteMsg=warning  WriteAfterReadMsg=warning  ShowAdditionalParam=off
  Data Store Memory7 : DataStoreMemory  DataStoreName=vzk5  ReadBeforeWriteMsg=warning  WriteAfterWriteMsg=warning  WriteAfterReadMsg=warning  ShowAdditionalParam=off
  Data Store Memory8 : DataStoreMemory  DataStoreName=xyk50  ReadBeforeWriteMsg=warning  WriteAfterWriteMsg=warning  WriteAfterReadMsg=warning  ShowAdditionalParam=off
  Data Store Memory9 : DataStoreMemory  DataStoreName=xxk50  ReadBeforeWriteMsg=warning  WriteAfterWriteMsg=warning  WriteAfterReadMsg=warning  ShowAdditionalParam=off
  Data Store Read : DataStoreRead  DataStoreName=count5  IndexOptions=Index vector (dialog)  Indices=1  OutputSizes=1
  Data Store Read1 : DataStoreRead  DataStoreName=xxk5  IndexOptions=Index vector (dialog)  Indices=1  OutputSizes=1
  Data Store Read10 : DataStoreRead  DataStoreName=vxk50  IndexOptions=Index vector (dialog)  Indices=1  OutputSizes=1
  Data Store Read11 : DataStoreRead  DataStoreName=vyk50  IndexOptions=Index vector (dialog)  Indices=1  OutputSizes=1
  Data Store Read12 : DataStoreRead  DataStoreName=vzk50  IndexOptions=Index vector (dialog)  Indices=1  OutputSizes=1
  Data Store Read2 : DataStoreRead  DataStoreName=xyk5  IndexOptions=Index vector (dialog)  Indices=1  OutputSizes=1
  Data Store Read3 : DataStoreRead  DataStoreName=xzk5  IndexOptions=Index vector (dialog)  Indices=1  OutputSizes=1
  Data Store Read4 : DataStoreRead  DataStoreName=vxk5  IndexOptions=Index vector (dialog)  Indices=1  OutputSizes=1
  Data Store Read5 : DataStoreRead  DataStoreName=vyk5  IndexOptions=Index vector (dialog)  Indices=1  OutputSizes=1
  Data Store Read6 : DataStoreRead  DataStoreName=vzk5  IndexOptions=Index vector (dialog)  Indices=1  OutputSizes=1
  Data Store Read7 : DataStoreRead  DataStoreName=xxk50  IndexOptions=Index vector (dialog)  Indices=1  OutputSizes=1
  Data Store Read8 : DataStoreRead  DataStoreName=xyk50  IndexOptions=Index vector (dialog)  Indices=1  OutputSizes=1
  Data Store Read9 : DataStoreRead  DataStoreName=xzk50  IndexOptions=Index vector (dialog)  Indices=1  OutputSizes=1
  Data Store Write : DataStoreWrite  DataStoreName=count5  IndexOptions=Index vector (dialog)  Indices=1  OutputSizes=1
  Data Store Write1 : DataStoreWrite  DataStoreName=xxk5  IndexOptions=Index vector (dialog)  Indices=1  OutputSizes=1
  Data Store Write10 : DataStoreWrite  DataStoreName=vxk50  IndexOptions=Index vector (dialog)  Indices=1  OutputSizes=1
  Data Store Write11 : DataStoreWrite  DataStoreName=vyk50  IndexOptions=Index vector (dialog)  Indices=1  OutputSizes=1
  Data Store Write12 : DataStoreWrite  DataStoreName=vzk50  IndexOptions=Index vector (dialog)  Indices=1  OutputSizes=1
  Data Store Write2 : DataStoreWrite  DataStoreName=xyk5  IndexOptions=Index vector (dialog)  Indices=1  OutputSizes=1
  Data Store Write3 : DataStoreWrite  DataStoreName=xzk5  IndexOptions=Index vector (dialog)  Indices=1  OutputSizes=1
  Data Store Write4 : DataStoreWrite  DataStoreName=vxk5  IndexOptions=Index vector (dialog)  Indices=1  OutputSizes=1
  Data Store Write5 : DataStoreWrite  DataStoreName=vyk5  IndexOptions=Index vector (dialog)  Indices=1  OutputSizes=1
  Data Store Write6 : DataStoreWrite  DataStoreName=vzk5  IndexOptions=Index vector (dialog)  Indices=1  OutputSizes=1
  Data Store Write7 : DataStoreWrite  DataStoreName=xxk50  IndexOptions=Index vector (dialog)  Indices=1  OutputSizes=1
  Data Store Write8 : DataStoreWrite  DataStoreName=xyk50  IndexOptions=Index vector (dialog)  Indices=1  OutputSizes=1
  Data Store Write9 : DataStoreWrite  DataStoreName=xzk50  IndexOptions=Index vector (dialog)  Indices=1  OutputSizes=1
  Demux1 : Demux  Outputs=12
  Display : Display
  L+B : Subsystem
  MATLAB Function : MATLAB Function  TreatAsAtomicUnit=on
  MATLAB Function2 : MATLAB Function  TreatAsAtomicUnit=on
  MATLAB Function3 : MATLAB Function  TreatAsAtomicUnit=on
  Memory : Memory
  Mux1 : Mux  Inputs=3
  Mux2 : Mux  Inputs=3
  Mux3 : Mux  Inputs=12
  Mux4 : Mux  Inputs=12
  Product : Product
  Product1 : Product
  Subsystem1 : Subsystem
  Subsystem2 : Subsystem
  Subsystem3 : Subsystem
  Subsystem4 : Subsystem
  Subsystem5 : Subsystem
  Subsystem6 : Subsystem
  Subtract : Sum  Inputs=+-
  Switch : Switch  Criteria=u2 > Threshold
  Switch2 : Switch  Criteria=u2 > Threshold
  u5 : Outport
  wires:
  Bus Selector6/4 -> Subsystem4/4(vz)  "<vz>"
  Bus Selector6/3 -> Subsystem4/3(vzk)  "<vz>"
  Bus Selector6/2 -> Subsystem4/2(xz)  "<xz>"
  Bus Selector6/1 -> Subsystem4/1(xzk)  "<xz>"
  Bus Selector5/4 -> Subsystem3/4(vy)  "<vy>"
  Bus Selector5/3 -> Subsystem3/3(vyk)  "<vy>"
  Bus Selector5/2 -> Subsystem3/2(xy)  "<xy>"
  Bus Selector5/1 -> Subsystem3/1(xyk)  "<xy>"
  Bus Selector4/4 -> Subsystem1/4(vx)  "<vx>"
  Bus Selector4/3 -> Subsystem1/3(vxk)  "<vx>"
  Bus Selector4/2 -> Subsystem1/2(xx)  "<xx>"
  Bus Selector4/1 -> Subsystem1/1(xxk)  "<xx>"
  Memory/1 -> u5/1  "node5"
  Product/1 -> Subtract/2
  Switch2/1 -> Add/1  "e1"
  MATLAB Function3/1(y) -> Product1/2
  Constant5/1 -> Switch2/3
  Constant/1 -> Product/2
  Constant4/1 -> Switch2/1
  MATLAB Function2/1(y) -> Product1/1
  L+B/1(u) -> MATLAB Function3/1(u)
  Mux1/1 -> MATLAB Function2/1(u)
  Subsystem4/1(ez) -> Mux1/3
  Subsystem1/1(ex) -> Mux1/1
  Add/1 -> Display/1, Data Store Write/1
  Product1/1 -> Subtract/1
  Mux2/1 -> MATLAB Function/1(u)
  MATLAB Function/1(y) -> Product/1
  Subsystem3/1(ey) -> Mux1/2
  Data Store Read/1 -> Add/2
  Subsystem2/1(uty) -> Mux2/2
  Subsystem6/1(utx) -> Mux2/1
  Subsystem5/1(utz) -> Mux2/3
  Subtract/1 -> Switch2/2, Switch/2
  Data Store Read7/1 -> Mux3/7
  Demux1/4 -> Data Store Write4/1, Bus Creator3/4  "vx"
  Demux1/10 -> Data Store Write10/1, Bus Creator3/10  "vx0"
  Bus Selector7/3 -> Mux4/3  "<xz>"
  Bus Selector7/9 -> Mux4/9  "<xz>"
  Bus Selector7/6 -> Mux4/6  "<vz>"
  Bus Selector7/4 -> Mux4/4  "<vx>"
  Bus Selector7/7 -> Mux4/7  "<xx>"
  Data Store Read12/1 -> Mux3/12
  Demux1/6 -> Data Store Write6/1, Bus Creator3/6  "vz"
  Bus Selector7/1 -> Mux4/1  "<xx>"
  Bus Selector7/8 -> Mux4/8  "<xy>"
  Data Store Read10/1 -> Mux3/10
  Mux3/1 -> Switch/3
  Demux1/12 -> Data Store Write12/1, Bus Creator3/12  "vz0"
  Demux1/7 -> Data Store Write7/1, Bus Creator3/7  "xx0"
  Bus Selector7/2 -> Mux4/2  "<xy>"
  Demux1/9 -> Data Store Write9/1, Bus Creator3/9  "xz0"
  Demux1/2 -> Data Store Write2/1, Bus Creator3/2  "xy"
  Demux1/5 -> Data Store Write5/1, Bus Creator3/5  "vy"
  Data Store Read8/1 -> Mux3/8
  Bus Creator3/1 -> Memory/1
  Demux1/8 -> Data Store Write8/1, Bus Creator3/8  "xy0"
  Data Store Read11/1 -> Mux3/11
  Data Store Read1/1 -> Mux3/1
  Demux1/1 -> Data Store Write1/1, Bus Creator3/1  "xx"
  Data Store Read2/1 -> Mux3/2
  Demux1/11 -> Data Store Write11/1, Bus Creator3/11  "vy0"
  Data Store Read9/1 -> Mux3/9
  Data Store Read4/1 -> Mux3/4
  Mux4/1 -> Switch/1
  Data Store Read3/1 -> Mux3/3
  Bus Selector7/5 -> Mux4/5  "<vy>"
  Data Store Read5/1 -> Mux3/5
  Data Store Read6/1 -> Mux3/6
  Demux1/3 -> Data Store Write3/1, Bus Creator3/3  "xz"
  Switch/1 -> Demux1/1
  [state] -> Bus Selector7/1
  Bus Selector7/10 -> Mux4/10  "<vx>"
  Bus Selector7/11 -> Mux4/11  "<vy>"
  Bus Selector7/12 -> Mux4/12  "<vz>"
  Bus Selector1/6 -> Subsystem2/6(vy0)  "<vy0>"
  Bus Selector1/7 -> Subsystem2/7(vy3)  "<vy>"
  Bus Selector/8 -> Subsystem6/8(vx4)  "<vx>"
  Bus Selector2/3 -> Subsystem5/3(xz3)  "<xz>"
  Bus Selector1/2 -> Subsystem2/2(xy0)  "<xy0>"
  Bus Selector/6 -> Subsystem6/6(vx0)  "<vx0>"
  Bus Selector2/1 -> Subsystem5/1(xz5)  "<xz>"
  Bus Selector2/5 -> Subsystem5/5(vz5)  "<vz>"
  Bus Selector2/2 -> Subsystem5/2(xz0)  "<xz0>"
  Bus Selector1/1 -> Subsystem2/1(xy5)  "<xy>"
  Bus Selector/1 -> Subsystem6/1(xx5)  "<xx>"
  Bus Selector2/4 -> Subsystem5/4(xz4)  "<xz>"
  Bus Selector1/3 -> Subsystem2/3(xy3)  "<xy>"
  Bus Selector/3 -> Subsystem6/3(xx3)  "<xx>"
  Bus Selector/2 -> Subsystem6/2(xx0)  "<xx0>"
  In19/1 -> Bus Selector/1, Bus Selector2/1, [state], Bus Selector1/1, Bus Selector4/1, Bus Selector5/1, Bus Selector6/1
  Bus Selector1/4 -> Subsystem2/4(xy4)  "<xy>"
  Bus Selector1/8 -> Subsystem2/8(vy4)  "<vy>"
  Bus Selector/7 -> Subsystem6/7(vx3)  "<vx>"
  Bus Selector/4 -> Subsystem6/4(xx4)  "<xx>"
  Bus Selector/5 -> Subsystem6/5(vx5)  "<vx>"
  Bus Selector1/5 -> Subsystem2/5(vy5)  "<vy>"
  Bus Selector2/8 -> Subsystem5/8(vz4)  "<vz>"
  Bus Selector2/7 -> Subsystem5/7(vz3)  "<vz>"
  Bus Selector2/6 -> Subsystem5/6(vz0)  "<vz0>"
